simulink model "Rakete"  (R2017b)
settings: Solver=VariableStepAuto  StartTime=0.0  StopTime=900  RelTol=1e-3
settings Model: Creator=aby032  LastModifiedBy=aby032

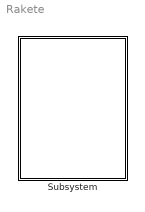
== system Rakete ==
  Subsystem : Subsystem  mask{m1_leer=500, m2_leer=1000, St1_Treibstoff=4000, St2_Treibstoff=1500, Durchsatz_1=20, Durchsatz_2=15, SchubProDurchsatz=4000}

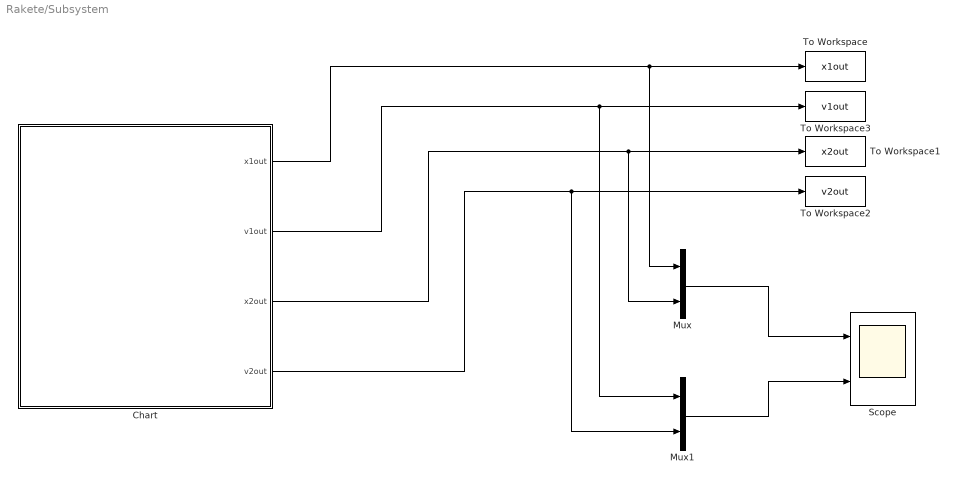
== system Rakete/Subsystem ==
  Chart : Stateflow chart  TreatAsAtomicUnit=on
  Mux : Mux  Inputs=2
  Mux1 : Mux  Inputs=2
  Scope : Scope  NumInputPorts=2
  To Workspace : ToWorkspace  VariableName=x1out  SaveFormat=Timeseries  SampleTime=-1
  To Workspace1 : ToWorkspace  VariableName=x2out  SaveFormat=Timeseries  SampleTime=-1
  To Workspace2 : ToWorkspace  VariableName=v2out  SaveFormat=Timeseries  SampleTime=-1
  To Workspace3 : ToWorkspace  VariableName=v1out  SaveFormat=Timeseries  SampleTime=-1
  wires:
  Mux1/1 -> Scope/2
  Chart/2(v1out) -> Mux1/1, To Workspace3/1
  Chart/4(v2out) -> Mux1/2, To Workspace2/1
  Chart/3(x2out) -> Mux/2, To Workspace1/1
  Chart/1(x1out) -> Mux/1, To Workspace/1
  Mux/1 -> Scope/1

== stateflow chart Rakete/Subsystem/Chart ==
  settings: updateMethod=CONTINUOUS
  state StufenGemeinsam
    during:
    %Derivatives
    [v1_dot,v2_dot]=Acc1();
    x1_dot=v1;
    x2_dot=v2;
    m1_dot=-Durchsatz_1;
    m2_dot=0;
    %Output
    x1out=x1;
    x2out=x2;
    v1out=v1;
    v2out=v2;
  state StufenGetrennt
    during:
    %Derivatives
    [v1_dot,v2_dot]=Acc2();
    x1_dot=v1;
    x2_dot=v2;
    m1_dot=0;
    m2_dot=-Durchsatz_2;
    %Output
    x1out=x1;
    x2out=x2;
    v1out=v1;
    v2out=v2;
  state Stufe2Ausgebrannt_
    during:
    %Derivatives
    [v1_dot,v2_dot]=Acc3();
    x1_dot=v1;
    x2_dot=v2;
    m1_dot=0;
    m2_dot=0;
    %Output
    x1out=x1;
    x2out=x2;
    v1out=v1;
    v2out=v2;
  (default) -> StufenGemeinsam : {Init()}
  StufenGetrennt -> Stufe2Ausgebrannt_ : [m2<=m2_leer]
  StufenGemeinsam -> StufenGetrennt : [m1<=m1_leer]
  data: a1 function_output; a2 function_output; a1 function_output; a2 function_output; a1 function_output; a2 function_output; x1out output double; v1out output double; x2out output double; v2out output double; m1_leer parameter double; m2_leer parameter double; St1_Treibstoff parameter double; St2_Treibstoff parameter double; Durchsatz_1 parameter double; Durchsatz_2 parameter double; SchubProDurchsatz parameter double; x1 local double; v1 local double; x2 local double; v2 local double; m1 local double; m2 local double; mE constant double =5.9736*10^24; rE constant double =6378000; G constant double =66.743*10^(-12)
  data x1 settings: updateMethod=SF_CONTINUOUS_TIME_DATA
  data v1 settings: updateMethod=SF_CONTINUOUS_TIME_DATA
  data x2 settings: updateMethod=SF_CONTINUOUS_TIME_DATA
  data v2 settings: updateMethod=SF_CONTINUOUS_TIME_DATA
  data m1 settings: updateMethod=SF_CONTINUOUS_TIME_DATA
  data m2 settings: updateMethod=SF_CONTINUOUS_TIME_DATA
  function Init:
    | function Init
    |     x1 = 0;
    |     v1 = 0;
    |     x2 = 0;
    |     v2 = 0;
    |     m1 = m1_leer + St1_Treibstoff;
    |     m2 = m2_leer + St2_Treibstoff;
    | end
  function [a1, a2]=Acc1:
    | function [a1, a2]=Acc1
    |  mR = m1 + m2;
    |  r = rE + x1;
    |  
    |  Fg = G*(mE*mR)/(r^2)                   %Endanziehungskraft auf die gesamte Rakete
    |  Fs = SchubProDurchsatz*Durchsatz_1;    %Schubkraft von der ersten Stuffe
    |  
    |  a1=(Fs-Fg)/mR;                         %Beschleunigung ist gleich da beide Stuffen verbunden
    |  a2=(Fs-Fg)/mR;
    | end
  function [a1, a2] = Acc2:
    | function [a1, a2] = Acc2
    |  r1 = rE + x1;                          %Abstand Erde - Stufe 1
    |  r2 = rE + x2;                          %Abstand Erde - Stufe 2
    |  
    |  Fg1 = G*(mE*m1)/(r1^2)                 %Endanziehungskraft auf Stufe 1
    |  Fg2 = G*(mE*m2)/(r2^2)                 %Endanziehungskraft auf Stufe 1
    |  
    |  Fs = SchubProDurchsatz*Durchsatz_2;    %Schubkraft von der zweiten Stufe
    |  
    |  
    |  a1=(-Fg1)/m1;                          %Beschleunigung Stufe 1
    |  a2=(Fs-Fg2)/m2;                        %Beschleunigung Stufe 2
    | end
  function [a1, a2] = Acc3:
    | function [a1, a2] = Acc3
    |  r1 = rE + x1;                          %Abstand Erde - Stufe 1
    |  r2 = rE + x2;                          %Abstand Erde - Stufe 2
    |  
    |  Fg1 = G*(mE*m1)/(r1^2)                 %Endanziehungskraft auf Stufe 1
    |  Fg2 = G*(mE*m2)/(r2^2)                 %Endanziehungskraft auf Stufe 
    |  
    |  a1=(-Fg1)/m1;                          %Beschleunigung Stufe 1
    |  a2=(-Fg2)/m2;                        %Beschleunigung Stufe 2
    | end
